simulink model "UDP_debug"  (R2023a)
settings: Solver=FixedStepAuto  StartTime=0.0  StopTime=inf  FixedStep=1e-4  RelTol=1e-3
undefined symbols (not defined in the file): f
libraries: instrumentlib x2, sldrtlib x1, realtime_pacer_lib x1
settings Model: Creator=xueji  LastModifiedBy=xueji

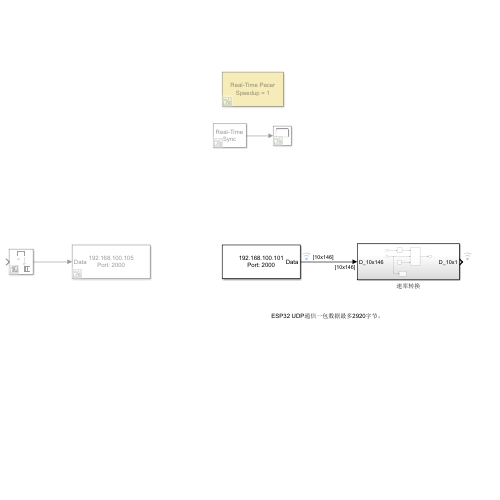
[thumbnail: Simulink's stored preview of the top-level diagram]
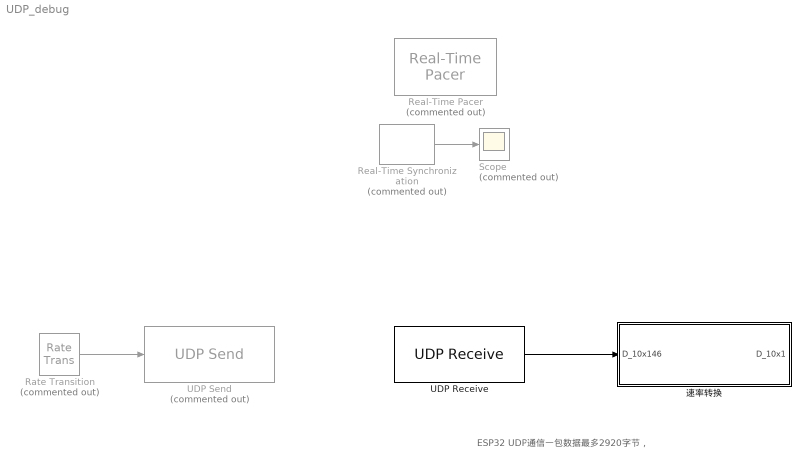
== system UDP_debug ==
  note: ESP32 UDP通信一包数据最多2920字节，
  Rate Transition : RateTransition  Commented=on  OutPortSampleTime=0.05
  Real-Time Synchronization : sldrtlib/Real-Time Synchronization  Commented=on  SampleTime=0.001  MaxMissedTicks=inf  ShowMissedTicks=on  YieldWhenWaiting=off
  Real-Time Pacer : realtime_pacer_lib/Real-Time Pacer  Commented=on  simTimePerRealTime=1
      settings: SourceProductName=Real-Time Pacer
  Scope : Scope  Commented=on
  UDP Receive : instrumentlib/UDP Receive  LocalAddress=192.168.100.101  LocalPort=2000  EnablePortSharing=off  Host=192.168.100.105  Port=2000  GetLatestData=on  DataSize=[10 146]  DataType=int16  ASCIIFormatting=%f,  Terminator=LF  CustomTerminator=10  ByteOrder=little-endian  EnableBlockingMode=on  Timeout=30  SampleTime=0.0146  SimulateUsing=Interpreted execution
  UDP Send : instrumentlib/UDP Send  Commented=on  Host=192.168.100.105  Port=2000  LocalAddress=192.168.100.101  LocalPort=2000  EnablePortSharing=off  OutputDatagramPacketSize=10  ByteOrder=little-endian  EnableBlockingMode=on  SimulateUsing=Interpreted execution
  速率转换 : Subsystem
  wires:
  Real-Time Synchronization/1 -> Scope/1
  Rate Transition/1 -> UDP Send/1
  UDP Receive/1 -> 速率转换/1(D_10x146)

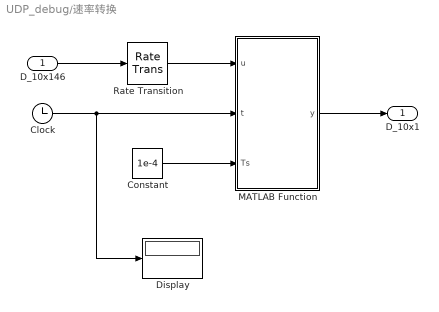
== system UDP_debug/速率转换 ==
  D_10x146 : Inport
  Clock : Clock
  Constant : Constant  Value=1e-4
  Display : Display
  MATLAB Function : MATLAB Function  TreatAsAtomicUnit=on
  Rate Transition : RateTransition
  D_10x1 : Outport
  wires:
  D_10x146/1 -> Rate Transition/1
  Rate Transition/1 -> MATLAB Function/1(u)
  Clock/1 -> Display/1, MATLAB Function/2(t)
  MATLAB Function/1(y) -> D_10x1/1
  Constant/1 -> MATLAB Function/3(Ts)

== matlab function UDP_debug/速率转换/MATLAB Function ==
  data: u input; y output; t input; Ts input
function y  = fcn(u,t,Ts)
    y = u(:,mod(int32(t/Ts),146)+1);
end
